simulink model "sampleModel1575"  (R2023a)
settings: Solver=VariableStepAuto  StartTime=0.0  StopTime=10.0  RelTol=1e-3
libraries: simulink x2, hdlsllib x2
settings Model: Creator=user1  LastModifiedBy=user1

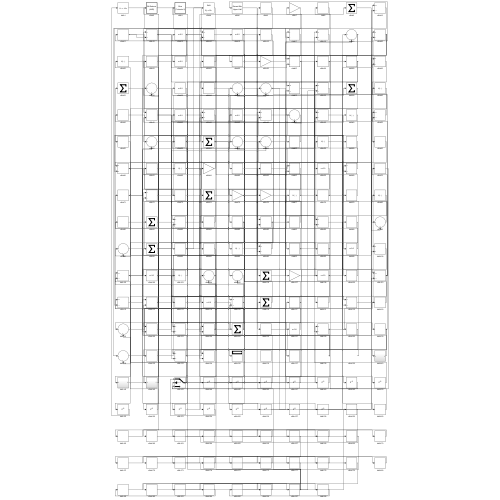
[thumbnail: Simulink's stored preview of the top-level diagram]
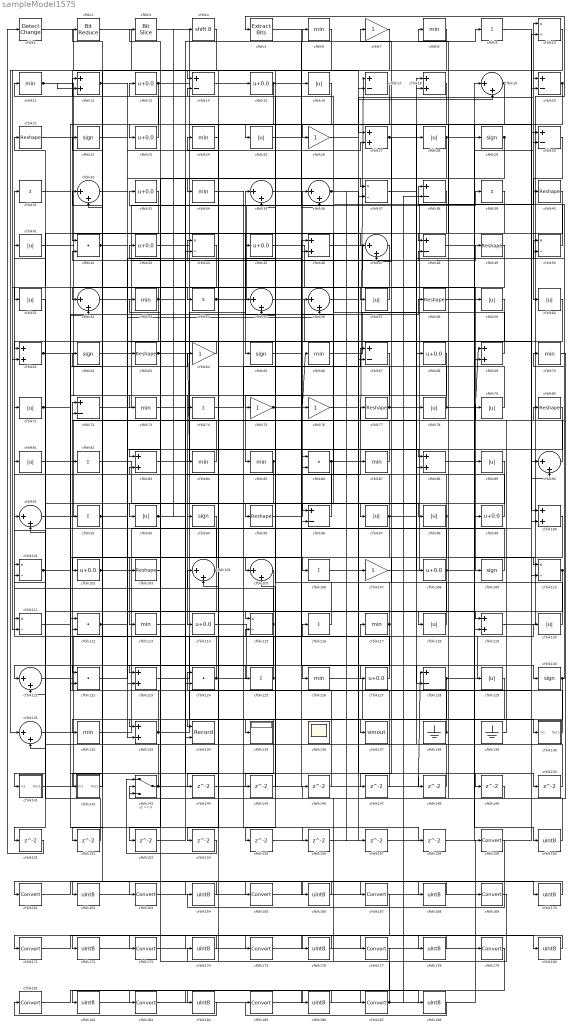
== system sampleModel1575 ==
  cfblk1 : simulink/Logic and Bit Operations/Detect Change  vinit=0  OutDataTypeStr=boolean
      settings: LibrarySourceBlock=|
      | hdlsllib/Logic and Bit
      | Operations/Detect
      | Change
  cfblk{10,37,44,50,101,110..111,115} (8 alike) : Product  Inputs=*/  RndMeth=Zero  SaturateOnIntegerOverflow=on
  cfblk{12,18,27,46,61,69,83,88,100,119,123,133} (12 alike) : Sum
  cfblk{13,15,23,33,43,45,68,99,102,108,114,127} (12 alike) : Bias  Bias=0.0  SaturateOnIntegerOverflow=off
  cfblk{21,40,49,58,63,77,80,95,103} (9 alike) : Reshape
  cfblk{19,32,35..36,47,52,55..56,90..91,104..105,121,131} (14 alike) : Sum  Inputs=|++
  cfblk{9,31,39,54,74,82,92,106,116,125} (10 alike) : Sum  Inputs=+
  cfblk{7,26,64,75..76,107} (6 alike) : Gain
  cfblk{22,29,62,65,94,109,130} (7 alike) : Signum
  cfblk{6,8,11,24,34,53,66,70,73,84..85,87,113,117,126,132} (16 alike) : MinMax
  cfblk{42,86,112,122,124} (5 alike) : DotProduct  OutDataTypeStr=Inherit: Inherit via internal rule
  cfblk{16,25,28,41,51,57,59..60,71,78..79,81,89,93,97..98,118,120,129} (19 alike) : Abs  SaturateOnIntegerOverflow=off
  cfblk{14,17,20,30,38,48,67,72,96,128} (10 alike) : Sum  Inputs=+-
  cfblk134 : Record  FileSettingsInternal="{\"entries\":[{\"content\":{\"excelSettings\":{\"content\":{},\"type\":\"Streamout.ExcelSettings\"}},\"type\":\"Streamout.FileSettingStorage\",\"uuid\":\"\"}],\"packageUris\":[\"http:\\/\\/schema.mathworks.com\\/mf0\\/streamout_blocks\\/R2020a\"],\"version\":\"1.0\"}"  Layout=[1 1]  SignalsInternal="{\"entries\":[{\"content\":{\"signals\":[{\"content\":{\"blockPath\":[],\"dimensions\":[1],\"domain\":\"\",\"lineColor\":\"#a2142f\",\"plots\":[1],\"port\":1,\"signalID\":1904,\"signalName\":\"XY Graph:1\"},\"type\":\"RecordBlkView.Signal\",\"uuid\":\"\"},{\"content\":{\"blockPath\":[],\"dimensions\":[1],\"domain\":\"\",\"lineColor\":\"#139fff\",\"plots\":[1],\"port\":2,\"signalID\":1907,\"signalName\":\"XY Graph:2\"},\"type\":\"RecordBlkView.Signal\",\"uuid\":\"\"}]},\"type\":\"RecordBlkView.InputSignals\",\"uuid\":\"\"}],\"packageUris\":[\"http:\\/\\/schema.mathworks.com\\/mf0\\/streamout_blocks\\/R2020a\"],\"version\":\"1.0\"}"  VisualizationBindings="{\"xyplotplugin\":{\"info\":[{\"series\":[{\"bindingParametersList\":[{\"parameter\":\"X-Axis\",\"signalID\":1904,\"signalName\":\"XY Graph:1\"},{\"parameter\":\"Y-Axis\",\"signalID\":1907,\"signalName\":\"XY Graph:2\"}],\"seriesID\":52600}],\"subplotID\":1}]}}"  CompatibilityTag=XY  st=-1
  cfblk135 : Display
  cfblk136 : Scope
      settings: Floating=on
  cfblk137 : ToWorkspace  VariableName=simout  SaveFormat=Timeseries  SampleTime=-1
  cfblk138 : Ground
  cfblk139 : Ground
  cfblk140 : Subsystem
      settings: LibrarySourceBlock=|
      | hdlsllib/Ports &
      | Subsystems/Subsystem
  cfblk141 : Subsystem
      settings: LibrarySourceBlock=|
      | hdlsllib/Ports &
      | Subsystems/Subsystem
  cfblk142 : Subsystem
      settings: LibrarySourceBlock=|
      | hdlsllib/Ports &
      | Subsystems/Subsystem
  cfblk143 : Switch  SaturateOnIntegerOverflow=off  InputSameDT=off
  cfblk{144..158} (15 alike) : Delay  SampleTime=1
  cfblk{159,161,163,165,167,169,171,173,175,177,179,181,183,185,187} (15 alike) : DataTypeConversion  SaturateOnIntegerOverflow=off  RndMeth=Floor
  cfblk{160,162,164,166,168,170,172,174,176,178,180,182,184,186,188} (15 alike) : DataTypeConversion  OutDataTypeStr=uint8  SaturateOnIntegerOverflow=off  RndMeth=Floor
  cfblk2 : hdlsllib/Logic and Bit Operations/Bit Reduce  mode=AND
  cfblk3 : hdlsllib/Logic and Bit Operations/Bit Slice  lidx=7  ridx=0
  cfblk4 : ArithShift  BitShiftNumber=8
  cfblk5 : simulink/Logic and Bit Operations/Extract Bits  bitsToExtract=Upper half  numBits=8  bitIdxRange=[0 7]  outScalingMode=Preserve fixed-point scaling
      settings: LibrarySourceBlock=|
      | hdlsllib/Logic and Bit
      | Operations/Extract Bits
  wires:
  cfblk13/1 -> cfblk137/1, cfblk68/1, cfblk122/2
  cfblk21/1 -> cfblk54/1
  cfblk125/1 -> cfblk31/1, cfblk104/2
  cfblk143/1 -> cfblk111/1, cfblk22/1, cfblk37/2, cfblk128/1
  cfblk68/1 -> cfblk85/1
  cfblk83/1 -> cfblk35/1
  cfblk72/1 -> cfblk38/1
  cfblk53/1 -> cfblk39/1, cfblk52/1, cfblk132/1
  cfblk24/1 -> cfblk131/1
  cfblk95/1 -> cfblk36/1
  cfblk86/1 -> cfblk17/1, cfblk134/1
  cfblk10/1 -> cfblk111/2
  cfblk127/1 -> cfblk72/1
  cfblk79/1 -> cfblk24/1
  cfblk119/1 -> cfblk5/1
  cfblk44/1 -> cfblk102/1
  cfblk97/1 -> cfblk71/1, cfblk50/1, cfblk122/1
  cfblk69/1 -> cfblk33/1
  cfblk128/1 -> cfblk120/1, cfblk134/2
  cfblk61/1 -> cfblk73/1, cfblk149/1
  cfblk23/1 -> cfblk13/1
  cfblk40/1 -> cfblk93/1
  cfblk4/1 -> cfblk42/1
  cfblk28/1 -> cfblk29/1, cfblk133/1
  cfblk2/1 -> cfblk27/1
  cfblk105/1 -> cfblk121/1
  cfblk14/1 -> cfblk15/1
  cfblk6/1 -> cfblk135/1
  cfblk45/1 -> cfblk57/1
  cfblk98/1 -> cfblk56/1, cfblk147/1
  cfblk15/1 -> cfblk25/1, cfblk128/2
  cfblk120/1 -> cfblk12/1
  cfblk41/1 -> cfblk114/1
  cfblk140/1(Out1) -> cfblk112/2
  cfblk92/1 -> cfblk118/1, cfblk56/2
  cfblk80/1 -> cfblk94/1
  cfblk46/1 -> cfblk109/1
  cfblk107/1 -> cfblk10/1
  cfblk58/1 -> cfblk99/1
  cfblk75/1 -> cfblk66/1, cfblk48/2
  cfblk111/1 -> cfblk58/1
  cfblk18/1 -> cfblk23/1
  cfblk43/1 -> cfblk129/1
  cfblk26/1 -> cfblk20/1
  cfblk123/1 -> cfblk89/1
  cfblk121/1 -> cfblk63/1
  cfblk9/1 -> cfblk90/1
  cfblk11/1 -> cfblk47/1, cfblk12/2
  cfblk113/1 -> cfblk87/1
  cfblk141/1(Out1) -> cfblk117/1
  cfblk82/1 -> cfblk95/1
  cfblk52/1 -> cfblk49/1
  cfblk110/1 -> cfblk70/1, cfblk40/1, cfblk123/1, cfblk50/2
  cfblk108/1 -> cfblk41/1, cfblk133/2, cfblk30/2
  cfblk16/1 -> cfblk75/1
  cfblk90/1 -> cfblk72/2
  cfblk5/1 -> cfblk36/2
  cfblk20/1 -> cfblk48/1, cfblk34/1, cfblk119/2
  cfblk54/1 -> cfblk9/1, cfblk97/1
  cfblk138/1 -> cfblk124/1, cfblk105/2
  cfblk124/1 -> cfblk91/1, cfblk100/2
  cfblk117/1 -> cfblk126/1, cfblk45/1
  cfblk118/1 -> cfblk77/1
  cfblk63/1 -> cfblk84/1, cfblk96/2
  cfblk130/1 -> cfblk80/1, cfblk152/1, cfblk153/1
  cfblk47/1 -> cfblk42/2
  cfblk37/1 -> cfblk108/1
  cfblk67/1 -> cfblk115/1
  cfblk3/1 -> cfblk90/2
  cfblk64/1 -> cfblk61/1
  cfblk84/1 -> cfblk62/1
  cfblk50/1 -> cfblk11/1
  cfblk32/1 -> cfblk88/1
  cfblk57/1 -> cfblk44/1
  cfblk66/1 -> cfblk28/1
  cfblk78/1 -> cfblk69/1, cfblk55/1
  cfblk91/1 -> cfblk18/2
  cfblk93/1 -> cfblk6/1, cfblk4/1
  cfblk65/1 -> cfblk86/1
  cfblk59/1 -> cfblk91/2
  cfblk71/1 -> cfblk74/1, cfblk64/1
  cfblk139/1 -> cfblk79/1
  cfblk74/1 -> cfblk67/1
  cfblk38/1 -> cfblk65/1
  cfblk133/1 -> cfblk10/2, cfblk2/1
  cfblk48/1 -> cfblk110/1
  cfblk85/1 -> cfblk142/1(In1), cfblk155/1
  cfblk12/1 -> cfblk37/1, cfblk119/1
  cfblk116/1 -> cfblk81/1
  cfblk126/1 -> cfblk140/1(In1)
  cfblk29/1 -> cfblk105/1, cfblk124/2
  cfblk114/1 -> cfblk116/1
  cfblk102/1 -> cfblk30/1, cfblk130/1
  cfblk35/1 -> cfblk98/1
  cfblk115/1 -> cfblk131/2, cfblk101/1
  cfblk132/1 -> cfblk76/1
  cfblk94/1 -> cfblk113/1
  cfblk55/1 -> cfblk100/1
  cfblk36/1 -> cfblk88/2, cfblk157/1
  cfblk39/1 -> cfblk96/1
  cfblk99/1 -> cfblk7/1
  cfblk122/1 -> cfblk103/1
  cfblk62/1 -> cfblk46/2
  cfblk77/1 -> cfblk78/1, cfblk55/2
  cfblk60/1 -> cfblk83/1
  cfblk22/1 -> cfblk27/2
  cfblk19/1 -> cfblk26/1, cfblk32/2
  cfblk87/1 -> cfblk35/2
  cfblk104/1 -> cfblk53/1, cfblk123/2
  cfblk30/1 -> cfblk60/1
  cfblk56/1 -> cfblk107/1
  cfblk49/1 -> cfblk61/2
  cfblk106/1 -> cfblk19/2
  cfblk142/1(Out1) -> cfblk92/1
  cfblk131/1 -> cfblk86/2
  cfblk25/1 -> cfblk16/1
  cfblk42/1 -> cfblk69/2, cfblk125/1
  cfblk81/1 -> cfblk82/1
  cfblk33/1 -> cfblk51/1
  cfblk27/1 -> cfblk59/1, cfblk47/2
  cfblk103/1 -> cfblk3/1
  cfblk51/1 -> cfblk141/1(In1)
  cfblk7/1 -> cfblk17/2
  cfblk96/1 -> cfblk83/2
  cfblk112/1 -> cfblk127/1, cfblk32/1
  cfblk1/1 -> cfblk14/1
  cfblk109/1 -> cfblk21/1
  cfblk70/1 -> cfblk143/2
  cfblk101/1 -> cfblk106/1, cfblk52/2
  cfblk17/1 -> cfblk144/1
  cfblk144/1 -> cfblk46/1
  cfblk129/1 -> cfblk145/1
  cfblk145/1 -> cfblk115/2
  cfblk146/1 -> cfblk14/2
  cfblk147/1 -> cfblk112/1
  cfblk73/1 -> cfblk148/1
  cfblk148/1 -> cfblk18/1
  cfblk149/1 -> cfblk143/3
  cfblk76/1 -> cfblk150/1
  cfblk150/1 -> cfblk121/2
  cfblk89/1 -> cfblk151/1
  cfblk151/1 -> cfblk1/1
  cfblk152/1 -> cfblk101/2
  cfblk153/1 -> cfblk44/2
  cfblk100/1 -> cfblk154/1
  cfblk154/1 -> cfblk143/1
  cfblk155/1 -> cfblk67/2
  cfblk31/1 -> cfblk156/1
  cfblk156/1 -> cfblk19/1
  cfblk157/1 -> cfblk110/2
  cfblk34/1 -> cfblk158/1
  cfblk158/1 -> cfblk20/2
  cfblk88/1 -> cfblk160/1
  cfblk160/1 -> cfblk8/1
  cfblk8/1 -> cfblk162/1
  cfblk162/1 -> cfblk159/1
  cfblk159/1 -> cfblk164/1
  cfblk164/1 -> cfblk161/1
  cfblk161/1 -> cfblk166/1
  cfblk166/1 -> cfblk163/1
  cfblk163/1 -> cfblk168/1
  cfblk168/1 -> cfblk165/1
  cfblk165/1 -> cfblk170/1
  cfblk170/1 -> cfblk167/1
  cfblk167/1 -> cfblk172/1
  cfblk172/1 -> cfblk169/1
  cfblk169/1 -> cfblk174/1
  cfblk174/1 -> cfblk171/1
  cfblk171/1 -> cfblk176/1
  cfblk176/1 -> cfblk173/1
  cfblk173/1 -> cfblk178/1
  cfblk178/1 -> cfblk175/1
  cfblk175/1 -> cfblk180/1
  cfblk180/1 -> cfblk177/1
  cfblk177/1 -> cfblk182/1
  cfblk182/1 -> cfblk179/1
  cfblk179/1 -> cfblk184/1
  cfblk184/1 -> cfblk181/1
  cfblk185/1 -> cfblk187/1
  cfblk181/1 -> cfblk186/1
  cfblk186/1 -> cfblk183/1
  cfblk187/1 -> cfblk146/1, cfblk38/2, cfblk104/1, cfblk43/1
  cfblk183/1 -> cfblk188/1
  cfblk188/1 -> cfblk185/1

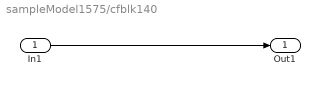
== system sampleModel1575/cfblk140 ==
  In1 : Inport
  Out1 : Outport
  wires:
  In1/1 -> Out1/1

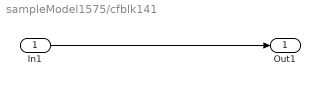
== system sampleModel1575/cfblk141 ==
  In1 : Inport
  Out1 : Outport
  wires:
  In1/1 -> Out1/1

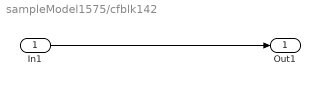
== system sampleModel1575/cfblk142 ==
  In1 : Inport
  Out1 : Outport
  wires:
  In1/1 -> Out1/1
